simulink model "tanks_closed"  (R2016a)
settings: Solver=VariableStepAuto  StartTime=0.0  StopTime=7.5  RelTol=1e-3
StartFcn:
  | global mdl;
  | mdl = run_setup;
settings Model: Creator=swsmth  LastModifiedBy=swsmth
settings GRTTargetCC: GeneratePreprocessorConditionals=Use local settings

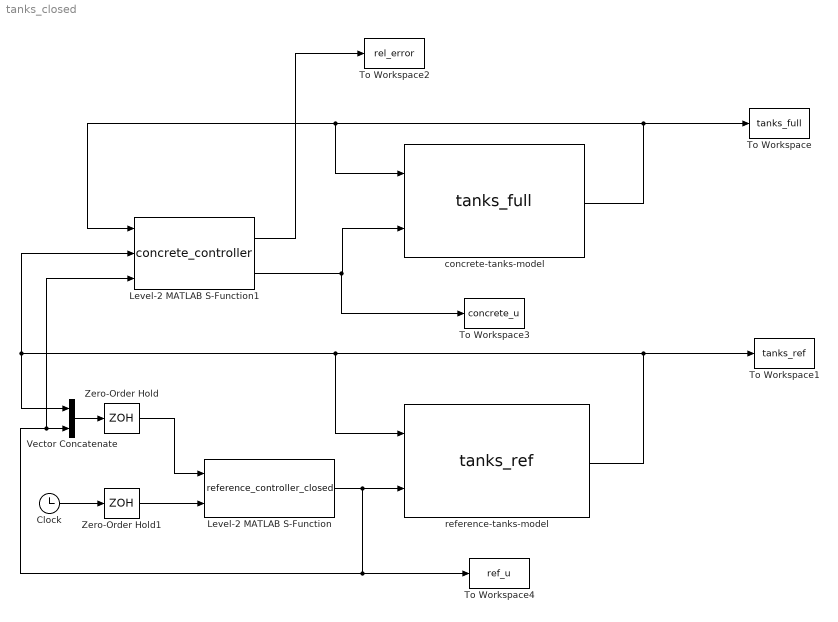
== system tanks_closed ==
  Clock : Clock
  Level-2 MATLAB S-Function : M-S-Function  FunctionName=reference_controller_closed
  Level-2 MATLAB S-Function1 : M-S-Function  FunctionName=concrete_controller
  To Workspace : ToWorkspace  VariableName=tanks_full  SampleTime=-1
  To Workspace1 : ToWorkspace  VariableName=tanks_ref  SampleTime=-1
  To Workspace2 : ToWorkspace  VariableName=rel_error  SampleTime=-1
  To Workspace3 : ToWorkspace  VariableName=concrete_u  SampleTime=-1
  To Workspace4 : ToWorkspace  VariableName=ref_u  SampleTime=-1
  Vector Concatenate : Concatenate
  Zero-Order Hold : ZeroOrderHold  SampleTime=.1
  Zero-Order Hold1 : ZeroOrderHold  SampleTime=.1
  concrete-tanks-model : M-S-Function  FunctionName=tanks_full
  reference-tanks-model : M-S-Function  FunctionName=tanks_ref
  wires:
  concrete-tanks-model/1 -> Level-2 MATLAB S-Function1/1, concrete-tanks-model/1, To Workspace/1
  reference-tanks-model/1 -> To Workspace1/1, reference-tanks-model/1, Level-2 MATLAB S-Function1/2, Vector Concatenate/1
  Zero-Order Hold/1 -> Level-2 MATLAB S-Function/1
  Level-2 MATLAB S-Function1/1 -> To Workspace2/1
  Level-2 MATLAB S-Function1/2 -> To Workspace3/1, concrete-tanks-model/2
  Level-2 MATLAB S-Function/1 -> Level-2 MATLAB S-Function1/3, Vector Concatenate/2, To Workspace4/1, reference-tanks-model/2
  Vector Concatenate/1 -> Zero-Order Hold/1
  Clock/1 -> Zero-Order Hold1/1
  Zero-Order Hold1/1 -> Level-2 MATLAB S-Function/2
